simulink model "reaction_pendulum_simulation"  (R2023b)
settings: Solver=FixedStepDiscrete  StartTime=0.0  StopTime=20  FixedStep=h  RelTol=1e-3  EnableMultiTasking=on
PreLoadFcn:
  | warning('off','MATLAB:dispatcher:InexactMatch');
InitFcn:
  | startup_sequence
StartFcn:
  | startup_sequence
model workspace (MAT data in the model file):
  square_freq = 0.5
values from neighbouring files (symbols this model uses):
  K_LQR = lqr(A,B,Q,R)    [LQR_gain.m]
  linearization_point = [0;0;0]    [startup_sequence.m]
  lp_deviation = [pi/9;0;0]    [startup_sequence.m]
  T = 0:h:T_f    [combi_input_signal.m]
undefined symbols (not defined in the file or in its folder): A_MPC_con, b_MPC_con, dim, H_nlobs, M_MPC, P_MPC, Q_MPC, R_MPC, S
settings Model: ExtModeTrigDuration=100000  Creator=user  LastModifiedBy=india
settings DataIOCC: SaveFormat=Array  SignalLoggingSaveFormat=ModelDataLogs  SaveOutput=off  SignalLogging=off  DSMLogging=off  SaveTime=off  ReturnWorkspaceOutputs=off
settings OptimizationCC: ExpressionDepthLimit=2147483647  LifeSpan=inf
settings DebuggingCC: UnderspecifiedInitializationDetection=Classic  MergeDetectMultiDrivingBlocksExec=none  SolverPrmCheckMsg=warning  FcnCallInpInsideContextMsg=warning  UnconnectedInputMsg=warning  UnconnectedOutputMsg=warning  UnconnectedLineMsg=warning  StateNameClashWarn=warning  SFUnexpectedBacktrackingDiag=warning  SFNoUnconditionalDefaultTransitionDiag=warning  SFExecutionAtInitializationDiag=none  ArithmeticOperatorsInVariantConditions=warning
settings HardwareCC: ProdBitPerPointer=32  ProdBitPerSizeT=32  ProdBitPerPtrDiffT=32  ProdLargestAtomicFloat=None  ProdIntDivRoundTo=Undefined  ProdEndianess=Unspecified  ProdWordSize=32  ProdHWDeviceType=32-bit Generic
settings ModelReferenceCC: EnableRefExpFcnMdlSchedulingChecks=on  PropagateSignalLabelsOutOfModel=off
settings SFSimCC: SimUseLocalCustomCode=off  CustomCodeUndefinedFunction=UseInterfaceOnly
settings RTWCC: Description=rpend RTDAC/USB2 (Visual C/C++)  SystemTargetFile=rtcon_rpend_usb2.tlc  TemplateMakefile=rtcon_rpend_vc_usb2_x64.tmf  RTWUseLocalCustomCode=off  DLArmComputeVersion=19.05
settings CodeAppCC: StateflowObjectComments=on
settings STFCustomTargetCC: TargetLangStandard=C89/C90 (ANSI)  ModelReferenceCompliant=off  CombineOutputUpdateFcns=on  MatFileLogging=on  SystemTargetFile=rtcon_rpend_usb2.tlc
settings GRTTargetCC: TargetLangStandard=C89/C90 (ANSI)  ModelReferenceCompliant=off  ParMdlRefBuildCompliant=off  CompOptLevelCompliant=off  ConcurrentExecutionCompliant=off  CPPClassGenCompliant=off  UseToolchainInfoCompliant=off  ExtMode=on  ExtModeMexFile=rtcon_ext_comm
settings ConfigComp: CovMetricSettings=dw  CovSaveCumulativeToWorkspaceVar=on  CovSaveSingleToWorkspaceVar=on  CovExternalEMLEnable=off  CovSFcnEnable=off

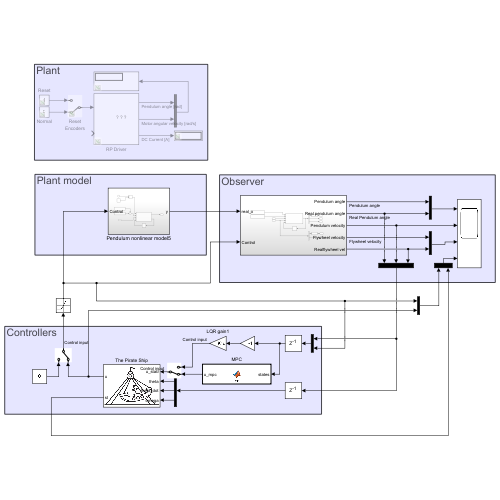
[thumbnail: Simulink's stored preview of the top-level diagram]
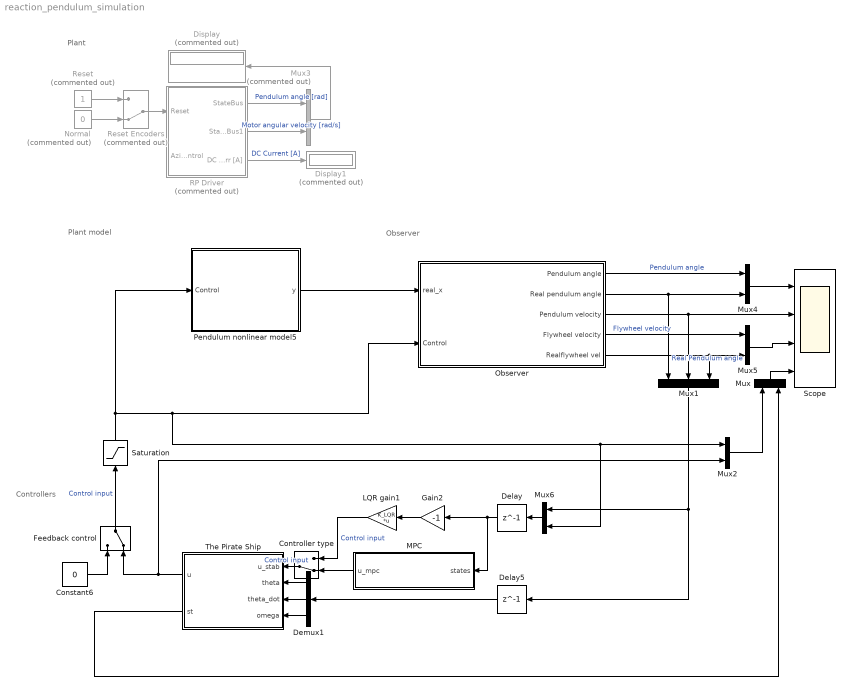
== system reaction_pendulum_simulation ==
  note: Plant model
  note: Controllers
  note: Observer
  note: Plant
  Constant6 : Constant  Value=0
  Controller type : ManualSwitch  CurrentSetting=0
  Delay : Delay  DelayLength=1
  Delay5 : Delay  DelayLength=1  InitialCondition=linearization_point - lp_deviation
  Demux1 : Demux  Outputs=3
  Display : Display  Commented=on
  Display1 : Display  Commented=on
  Feedback control : ManualSwitch  CurrentSetting=0
  Gain2 : Gain  Gain=-1
  LQR gain1 : Gain  Gain=K_LQR  Multiplication=Matrix(K*u)
  MPC : MATLAB Function  TreatAsAtomicUnit=on
  Mux{,2,4..6} (5 alike) : Mux  Inputs=2
  Mux1 : Mux  Inputs=3
  Mux3 : Mux  Commented=on  Inputs=2
  Normal : Constant  Commented=on  Value=0
  Observer : Subsystem
  Pendulum nonlinear model5 : Subsystem
  RP Driver : Subsystem  Commented=on
      mask Display: image(imread('rwp.JPG'))
  Reset : Constant  Commented=on
  Reset Encoders : ManualSwitch  Commented=on  CurrentSetting=0
  Saturation : Saturate  UpperLimit=1  LowerLimit=-1
  Scope : Scope  NumInputPorts=4
  The Pirate Ship : Stateflow chart  TreatAsAtomicUnit=on
  wires:
  Normal/1 -> Reset Encoders/2
  Reset/1 -> Reset Encoders/1
  Reset Encoders/1 -> RP Driver/1(Reset)
  RP Driver/1(StateBus) -> Mux3/1  "Pendulum angle [rad]"
  Feedback control/1 -> Saturation/1  "Control input"
  Mux4/1 -> Scope/1
  Mux5/1 -> Scope/3
  Constant6/1 -> Feedback control/1
  RP Driver/2(StateBus1) -> Mux3/2  "Motor angular velocity [rad/s]"
  Observer/3(Pendulum velocity) -> Scope/2, Mux1/2
  Observer/4(Flywheel velocity) -> Mux5/1  "Flywheel velocity"
  Observer/5(Realflywheel vel) -> Mux5/2, Mux1/3
  Mux3/1 -> Display/1
  Demux1/2 -> The Pirate Ship/3(theta_dot)
  Demux1/3 -> The Pirate Ship/4(omega)
  Demux1/1 -> The Pirate Ship/2(theta)
  Observer/1(Pendulum angle) -> Mux4/1  "Pendulum angle"
  Observer/2(Real pendulum angle) -> Mux1/1, Mux4/2  "Real Pendulum angle"
  Mux/1 -> Scope/4
  Delay5/1 -> Demux1/1
  Gain2/1 -> LQR gain1/1
  Controller type/1 -> The Pirate Ship/1(u_stab)  "Control input"
  Mux1/1 -> Mux6/1, Delay5/1
  MPC/1(u_mpc) -> Controller type/2
  LQR gain1/1 -> Controller type/1  "Control input"
  The Pirate Ship/1(u) -> Mux2/2, Feedback control/2
  The Pirate Ship/2(st) -> Mux/2
  RP Driver/3(DC Curr [A]) -> Display1/1  "DC Current [A]"
  Mux2/1 -> Mux/1
  Saturation/1 -> Pendulum nonlinear model5/1(Control), Mux6/2, Mux2/1, Observer/2(Control)
  Mux6/1 -> Delay/1
  Delay/1 -> MPC/1(states), Gain2/1
  Pendulum nonlinear model5/1(y) -> Observer/1(real_x)

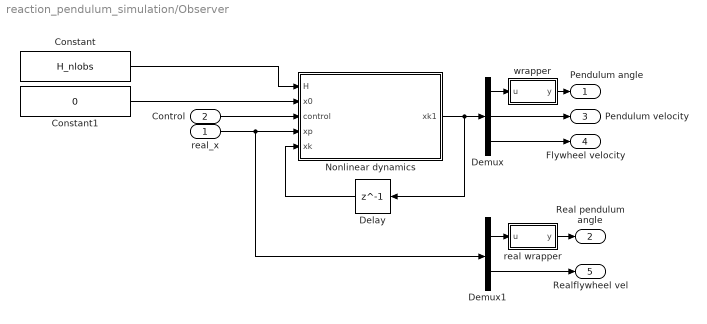
== system reaction_pendulum_simulation/Observer ==
  real_x : Inport
  Control : Inport  Port=2
  Constant : Constant  Value=H_nlobs
  Constant1 : Constant  Value=0
  Delay : Delay  DelayLength=1
  Demux : Demux  Outputs=3
  Demux1 : Demux  Outputs=2
  Nonlinear dynamics : MATLAB Function  TreatAsAtomicUnit=on
  real wrapper : MATLAB Function  TreatAsAtomicUnit=on
  wrapper : MATLAB Function  TreatAsAtomicUnit=on
  Pendulum angle : Outport
  Real pendulum angle : Outport  Port=2
  Pendulum velocity : Outport  Port=3
  Flywheel velocity : Outport  Port=4
  Realflywheel vel : Outport  Port=5
  wires:
  Delay/1 -> Nonlinear dynamics/5(xk)
  Control/1 -> Nonlinear dynamics/3(control)
  Nonlinear dynamics/1(xk1) -> Demux/1, Delay/1
  real_x/1 -> Demux1/1, Nonlinear dynamics/4(xp)
  Constant/1 -> Nonlinear dynamics/1(H)
  Constant1/1 -> Nonlinear dynamics/2(x0)
  Demux/2 -> Pendulum velocity/1
  Demux/3 -> Flywheel velocity/1
  Demux1/2 -> Realflywheel vel/1
  Demux/1 -> wrapper/1(u)
  wrapper/1(y) -> Pendulum angle/1
  Demux1/1 -> real wrapper/1(u)
  real wrapper/1(y) -> Real pendulum angle/1

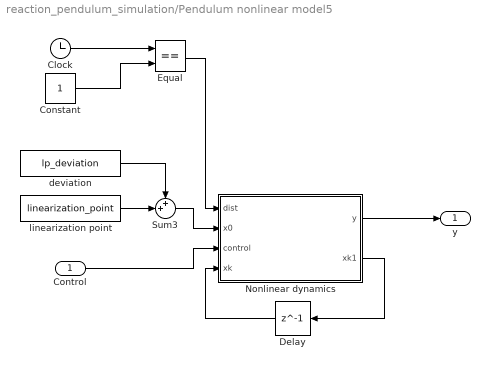
== system reaction_pendulum_simulation/Pendulum nonlinear model5 ==
  Control : Inport
  Clock : Clock
  Constant : Constant
  Delay : Delay  DelayLength=1
  Equal : RelationalOperator  Operator===  OutDataTypeStr=boolean  RndMeth=Simplest  InputSameDT=off
  Nonlinear dynamics : MATLAB Function  TreatAsAtomicUnit=on
  Sum3 : Sum  Inputs=++|
  deviation : Constant  Value=lp_deviation
  linearization point : Constant  Value=linearization_point
  y : Outport
  wires:
  Delay/1 -> Nonlinear dynamics/4(xk)
  Sum3/1 -> Nonlinear dynamics/2(x0)
  Control/1 -> Nonlinear dynamics/3(control)
  Nonlinear dynamics/2(xk1) -> Delay/1
  Nonlinear dynamics/1(y) -> y/1
  deviation/1 -> Sum3/1
  linearization point/1 -> Sum3/2
  Clock/1 -> Equal/1
  Constant/1 -> Equal/2
  Equal/1 -> Nonlinear dynamics/1(dist)

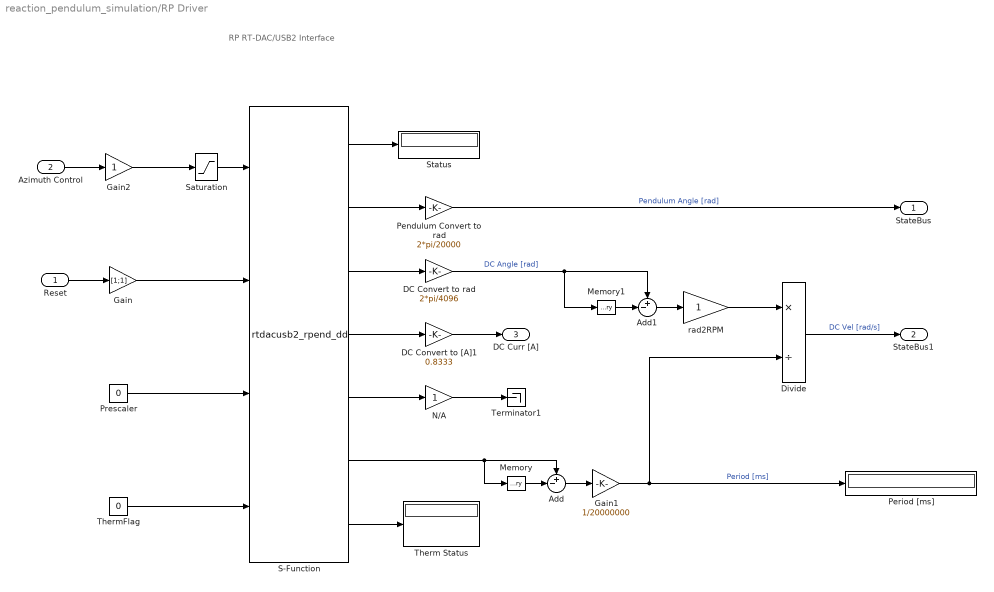
== system reaction_pendulum_simulation/RP Driver ==
  note: RP RT-DAC/USB2
      | Interface
  Reset : Inport
  Azimuth Control : Inport  Port=2
  Add : Sum  Inputs=+-|
  Add1 : Sum  Inputs=+-|
  DC Convert to [A]1 : Gain  Gain=0.8333  SaturateOnIntegerOverflow=on  OutDataTypeStr=Inherit: Same as input  ParamDataTypeStr=Inherit: Same as input
  DC Convert to rad : Gain  Gain=2*pi/4096  SaturateOnIntegerOverflow=on  OutDataTypeStr=Inherit: Same as input  ParamDataTypeStr=Inherit: Same as input
  Divide : Product  Inputs=*/
  Gain : Gain  Gain=[1;1]
  Gain1 : Gain  Gain=1/20000000
  Gain2 : Gain
  Memory : Memory
  Memory1 : Memory
  N/A : Gain  SaturateOnIntegerOverflow=on  OutDataTypeStr=Inherit: Same as input  ParamDataTypeStr=Inherit: Same as input
  Pendulum Convert to rad : Gain  Gain=2*pi/20000  SaturateOnIntegerOverflow=on  OutDataTypeStr=Inherit: Same as input  ParamDataTypeStr=Inherit: Same as input
  Period [ms] : Display
  Prescaler : Constant  Value=0
  S-Function : S-Function  FunctionName=rtdacusb2_rpend_dd  Parameters=1, h  SFunctionDeploymentMode=off  EnableBusSupport=off
  Saturation : Saturate  UpperLimit=1  LowerLimit=-1
  Status : Display
  Terminator1 : Terminator
  Therm Status : Display
  ThermFlag : Constant  Value=0
  rad2RPM : Gain  SaturateOnIntegerOverflow=on  OutDataTypeStr=Inherit: Same as input  ParamDataTypeStr=Inherit: Same as input
  StateBus : Outport  VectorParamsAs1DForOutWhenUnconnected=off
  StateBus1 : Outport  Port=2  VectorParamsAs1DForOutWhenUnconnected=off
  DC Curr [A] : Outport  Port=3  VectorParamsAs1DForOutWhenUnconnected=off
  wires:
  S-Function/7 -> Therm Status/1
  S-Function/5 -> N/A/1
  S-Function/4 -> DC Convert to [A]1/1
  ThermFlag/1 -> S-Function/4
  Prescaler/1 -> S-Function/3
  Gain/1 -> S-Function/2
  DC Convert to [A]1/1 -> DC Curr [A]/1
  Divide/1 -> StateBus1/1  "DC Vel [rad/s]"
  rad2RPM/1 -> Divide/1
  Add1/1 -> rad2RPM/1
  Memory1/1 -> Add1/2
  N/A/1 -> Terminator1/1
  S-Function/6 -> Add/1, Memory/1
  Gain2/1 -> Saturation/1
  Gain1/1 -> Period [ms]/1, Divide/2  "Period [ms]"
  Add/1 -> Gain1/1
  Memory/1 -> Add/2
  DC Convert to rad/1 -> Add1/1, Memory1/1  "DC Angle [rad]"
  S-Function/3 -> DC Convert to rad/1
  Pendulum Convert to rad/1 -> StateBus/1  "Pendulum Angle [rad]"
  S-Function/2 -> Pendulum Convert to rad/1
  S-Function/1 -> Status/1
  Saturation/1 -> S-Function/1
  Reset/1 -> Gain/1
  Azimuth Control/1 -> Gain2/1

== stateflow chart reaction_pendulum_simulation/The Pirate Ship ==
  state Swing_up
    u=-ku*sign(theta_dot);
    st = -0.1;
  state Nothing
    u=0;
    st = 0;
  state Slow_down
    u=kp*sign(theta_dot);
    st = 0.1;
  state Stabilizing
    u=u_stab;
    st=0.4;
  state Flywheel_limit
    u=0;
  Nothing -> Swing_up [order 1] : [abs(theta)>wheel]
  Swing_up -> Nothing : [abs(theta)<wheel]
  Nothing -> Slow_down [order 3] : [abs(theta)<pi/2 && abs(theta_dot)>vmax]
  Slow_down -> Nothing : [abs(theta_dot)<3/4*vmax]
  Nothing -> Stabilizing [order 2] : [abs(theta) < delta]
  Stabilizing -> Nothing [order 1] : [abs(theta) > delta]
  (default) -> Nothing
  Flywheel_limit -> Stabilizing : [abs(omega)<200]
  Stabilizing -> Flywheel_limit [order 2] : [abs(omega)>250]
  data: u_stab input; theta input; theta_dot input; u output; ku local =0.8; kp local =1; delta local =deg2rad(20); vmax local =5; wheel local =pi-deg2rad(60); st output; omega input

== matlab function reaction_pendulum_simulation/Observer/wrapper ==
  data: u input; y output
function y = fcn(u)

y = mod(u,2*pi)-pi;

end

== matlab function reaction_pendulum_simulation/Observer/real wrapper ==
  data: u input; y output
function y = fcn(u)

y = mod(u,2*pi)-pi;

end

== matlab function reaction_pendulum_simulation/MPC ==
  data: states input; u_mpc output; T parameter; S parameter; Q_MPC parameter; R_MPC parameter; dim parameter; P_MPC parameter; M_MPC parameter; A_MPC_con parameter; b_MPC_con parameter
function u_mpc = fcn(states, T,S,Q_MPC,R_MPC,dim,P_MPC,M_MPC,A_MPC_con, b_MPC_con)
    x0 = [states;0];
    [left,right]=costgen(T,S,Q_MPC,R_MPC,dim,x0,P_MPC,M_MPC);
    u0 = zeros(size(right));
%     u_mpc = 0;
    opts = optimoptions('quadprog','Display','off','Algorithm','active-set');
    u_N = quadprog(left,right,A_MPC_con,b_MPC_con,[],[],[],[],u0,opts);
    u_mpc = u_N(1);
end

function [H,h]=costgen(T,S,Q,R,dim,x0,P,M)
    % Cost function generation
    % Converts a cost function of the form:
    % V_N(x(0),u_n) = 0.5*sum_{0,N-1}(x'Qx + u'Ru + 2x'Mu) + 0.5x_N'Px_N
    % into a form only dependent on u_N:
    % V_N(u_N) = 0.5u'Hu + h'u + c
    
    if nargin == 6
        M = zeros(dim.nx,dim.nu);
        P = Q;
    end
    
    % Define the bar matrices Qbar, Rbar, Mbar
    Qbar = blkdiag(kron(eye(dim.N),Q),P); 
    Rbar = kron(eye(dim.N),R);
    Mbar = [kron(eye(dim.N),M);zeros(dim.nx,dim.N*dim.nu)];
    
    % Calculate H,h,c
    H = (Rbar + S'*Qbar*S + 2*S'*Mbar);  
    
    % Stabilizing version
    h = (S'*Qbar*T*x0 + Mbar'*T*x0);
end

== matlab function reaction_pendulum_simulation/Observer/Nonlinear dynamics ==
  data: H input; x0 input; control input; xp input; xk input size=[3,1]; xk1 output size=[3,1]; h parameter
function xk1   = nlrk4(H, x0, control, xp, xk, h)
    persistent initialized
    persistent initialized2

    if isempty(initialized)
        xk1 = [xp(1);x0;xp(2)];
        theta_dd = 0;
        initialized = true;
        return;
    end

    if isempty(initialized2)
        xk1 = [xp(1);x0;xp(2)];
        theta_dd = 0;
        initialized2 = true;
        return;
    end

    function dx = nlf(t,x,u,xp,H)
        C = [1,0,0;0,0,1];

        % Define constants
        K1 = 10.6608;
        K2 = 0.0487;
        K3 = 0.1031;
        K4 = 404.3827;
        K5 = 0.9442;
        K6 = 1.7125;
        K_tau = 0.0107;
        
        % System equations
        theta = x(1);
        theta_dot = x(2);
        omega = x(3);
        theta_ddot = -K1*sin(theta)-K2*theta_dot-K3*sign(theta_dot)-K_tau*(K4*u-K5*omega-K6*sign(omega));
        omega_dot = K4*u-K5*omega-K6*sign(omega);
        delta = xp-C*x;
        Linear_term = H*(delta);
        NL_term = [theta_dot; theta_ddot; omega_dot] ;
        dx = NL_term + Linear_term;
    end

    function theta_ddot = theta_ddd(t,x,u,xp,H)
        C = [1,0,0;0,0,1];

        % Define constants
        K1 = 10.6608;
        K2 = 0.0487;
        K3 = 0.1031;
        K4 = 404.3827;
        K5 = 0.9442;
        K6 = 1.7125;
        K_tau = 0.0107;
        
        % System equations
        theta = x(1);
        theta_dot = x(2);
        omega = x(3);
        theta_ddot = -K1*sin(theta)-K2*theta_dot-K3*sign(theta_dot)-K_tau*(K4*u-K5*omega-K6*sign(omega));
    end

    theta_dd = theta_ddd(0, xk, control, xp, H);

    % Executes one timestep of the RK4 algorithm
    k1 = nlf(0, xk, control, xp, H);
    k2 = nlf(0 + h/2, xk + h/2*k1, control, xp + h/2*k1([1,3]), H);
    k3 = nlf(0 + h/2, xk + h/2*k2, control, xp + h/2*k2([1,3]), H);
    k4 = nlf(0 + h, xk + h*k3, control, xp + h*k3([1,3]), H);
    xk1 = xk + h/6*(k1 + 2*k2 + 2*k3 + k4);

    % % Forward Euler
    % xk1 = xk + h*nlf(0, xk, control);
    % Take out states of interest
    % y = [xk(1); xk(3)];
end

== matlab function reaction_pendulum_simulation/Pendulum nonlinear model5/Nonlinear dynamics ==
  data: dist input; x0 input; y output; control input; xk input size=[3,1]; xk1 output size=[3,1]; h parameter
function [y, xk1] = nlrk4(dist, x0, control, xk, h)
    persistent initialized

    if isempty(initialized)
        xk = x0;
        initialized = true;
    end

    function dx = nlf(t,x,u)
    
        % Define constants
        K1 = 10.6608;
        K2 = 0.0487;
        K3 = 0.1031;
        K4 = 404.3827;
        K5 = 0.9442;
        K6 = 1.7125;
        K_tau = 0.0107;
        
        % System equations
        theta = x(1);
        theta_dot = x(2);
        omega = x(3);
        theta_ddot = -K1*sin(theta)-K2*theta_dot-K3*sign(theta_dot)-K_tau*(K4*u-K5*omega-K6*sign(omega));
        omega_dot = K4*u-K5*omega-K6*sign(omega);
        dx = [theta_dot; theta_ddot; omega_dot];
    end

    % Executes one timestep of the RK4 algorithm
    k1 = nlf(0, xk, control);
    k2 = nlf(0 + h/2, xk + h/2*k1, control);
    k3 = nlf(0 + h/2, xk + h/2*k2, control);
    k4 = nlf(0 + h, xk + h*k3, control);
    xk1 = xk + h/6*(k1 + 2*k2 + 2*k3 + k4);

    % if dist
    %     xk1(1)=pi/9;
    %     xk(1) = pi/9;
    % end

    % % Forward Euler
    % xk1 = xk + h*nlf(0, xk, control);
    % Take out states of interest
    y = [xk(1); xk(3)];
end
